simulink model "nxtLoopback"  (R2014b)
settings: Solver=FixedStepDiscrete  StartTime=0.0  StopTime=inf  FixedStep=0.1  RelTol=1e-3
InitFcn:
  | ben = comms.Bt(RobotID.NXT_BEN);
  | ben.init();
libraries: hostCommsLib x2, simulink x1
settings Model: Creator=nrattner  LastModifiedBy=ksurende

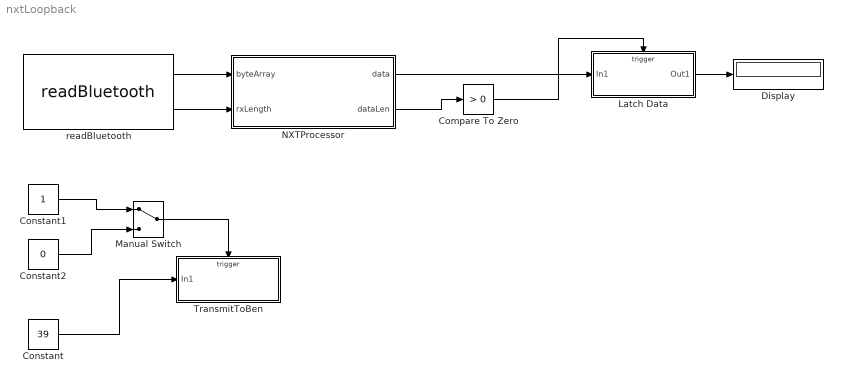
== system nxtLoopback ==
  Compare To Zero : simulink/Logic and Bit Operations/Compare To Zero  relop=>  OutDataTypeStr=boolean
  Constant : Constant  Value=39
  Constant1 : Constant  SampleTime=-1
  Constant2 : Constant  Value=0  SampleTime=-1
  Display : Display
  Latch Data : Subsystem  TreatAsAtomicUnit=on
  Manual Switch : ManualSwitch
  NXTProcessor : MATLAB Function  TreatAsAtomicUnit=on
  TransmitToBen : Subsystem  TreatAsAtomicUnit=on
  readBluetooth : hostCommsLib/readBluetooth  robotId=RobotID.NXT_BEN  numBytes=1
  wires:
  Compare To Zero/1 -> Latch Data/Trigger
  Constant/1 -> TransmitToBen/1(In1)
  readBluetooth/2 -> NXTProcessor/2(rxLength)
  NXTProcessor/2(dataLen) -> Compare To Zero/1
  NXTProcessor/1(data) -> Latch Data/1(In1)
  Manual Switch/1 -> TransmitToBen/Trigger
  Constant1/1 -> Manual Switch/1
  Constant2/1 -> Manual Switch/2
  Latch Data/1(Out1) -> Display/1
  readBluetooth/1 -> NXTProcessor/1(byteArray)

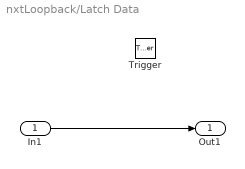
== system nxtLoopback/Latch Data ==
  In1 : Inport
  Trigger : TriggerPort
  Out1 : Outport
  wires:
  In1/1 -> Out1/1

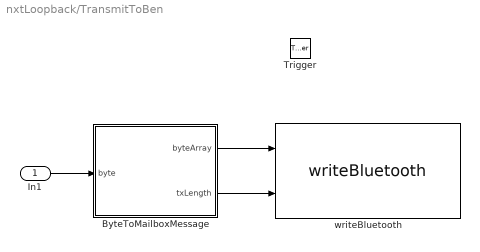
== system nxtLoopback/TransmitToBen ==
  In1 : Inport
  Trigger : TriggerPort  TriggerType=either
  ByteToMailboxMessage : MATLAB Function  TreatAsAtomicUnit=on
  writeBluetooth : hostCommsLib/writeBluetooth  robotId=RobotID.NXT_BEN
  wires:
  In1/1 -> ByteToMailboxMessage/1(byte)
  ByteToMailboxMessage/1(byteArray) -> writeBluetooth/1
  ByteToMailboxMessage/2(txLength) -> writeBluetooth/2

== matlab function nxtLoopback/TransmitToBen/ByteToMailboxMessage ==
  data: byte input; byteArray output; txLength output
function [byteArray,txLength] = fcn(byte)
%#codegen

byteArray = uint8([2 0 1 byte]);
txLength = 4;

== matlab function nxtLoopback/NXTProcessor ==
  data: data output; dataLen output; byteArray input uint8; rxLength input double
function [data,dataLen] = nxtProcessor(byteArray,rxLength)
%#codegen

persistent ben;

if(isempty(ben))
    bufferLen = uint8(1);
    ben = comms.RawNXTDataProcessor(bufferLen);
end

[data,dataLen] = ben.process(byteArray,uint8(rxLength));

end
